simulink model "JSON_TEST_2022"  (R2022a)
settings: Solver=VariableStepAuto  StartTime=0.0  StopTime=10.0  RelTol=1e-3
libraries: dspnetwork x1, instrumentlib x1
settings Model: Creator=santh  LastModifiedBy=santh
settings ModelReferenceCC: EnableRefExpFcnMdlSchedulingChecks=off
settings RTWCC: Description=Generic Real-Time Target  GPUComputeCapability=5.0

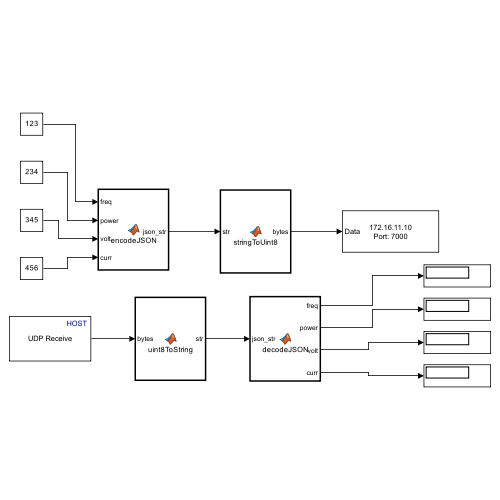
[thumbnail: Simulink's stored preview of the top-level diagram]
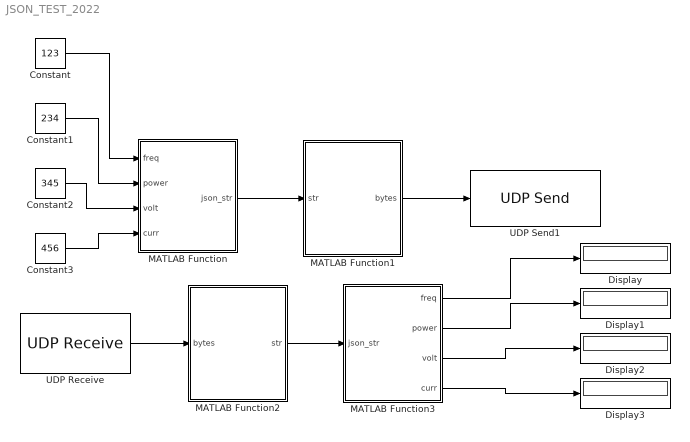
== system JSON_TEST_2022 ==
  Constant : Constant  Value=123
  Constant1 : Constant  Value=234
  Constant2 : Constant  Value=345
  Constant3 : Constant  Value=456
  Display{,1..3} (4 alike) : Display
  MATLAB Function : MATLAB Function  TreatAsAtomicUnit=on
  MATLAB Function1 : MATLAB Function  TreatAsAtomicUnit=on
  MATLAB Function2 : MATLAB Function  TreatAsAtomicUnit=on
  MATLAB Function3 : MATLAB Function  TreatAsAtomicUnit=on
  UDP Receive : dspnetwork/UDP Receive  localURL='0.0.0.0'  localPort=7000  remoteURL='172.16.11.10'  remotePort=-1  recvBufferSize=30  dims=64  signalDatatype=uint8  isComplex=off  isVarSize=on  showBlockingTime=on  blockingTime=0  sampletime=0.01  blockPlatform=HOST
  UDP Send1 : instrumentlib/UDP Send  Host=172.16.11.10  Port=7000  LocalAddress=176.16.11.69  LocalPort=7000  EnablePortSharing=off  OutputDatagramPacketSize=20  ByteOrder=BigEndian  EnableBlockingMode=on
  wires:
  Constant/1 -> MATLAB Function/1(freq)
  Constant1/1 -> MATLAB Function/2(power)
  Constant2/1 -> MATLAB Function/3(volt)
  Constant3/1 -> MATLAB Function/4(curr)
  MATLAB Function/1(json_str) -> MATLAB Function1/1(str)
  MATLAB Function1/1(bytes) -> UDP Send1/1
  UDP Receive/1 -> MATLAB Function2/1(bytes)
  MATLAB Function2/1(str) -> MATLAB Function3/1(json_str)
  MATLAB Function3/1(freq) -> Display/1
  MATLAB Function3/2(power) -> Display1/1
  MATLAB Function3/3(volt) -> Display2/1
  MATLAB Function3/4(curr) -> Display3/1

== matlab function JSON_TEST_2022/MATLAB Function1 ==
  data: str input; bytes output
function bytes = stringToUint8(str)
    bytes = uint8(char(str));
end

== matlab function JSON_TEST_2022/MATLAB Function ==
  data: freq input; json_str output; power input; volt input; curr input
function json_str = encodeJSON(freq, power, volt, curr)
    data = struct('frequency', freq, 'power', power, 'voltage', volt, 'current', curr);
    json_str = jsonencode(data);
end

== matlab function JSON_TEST_2022/MATLAB Function2 ==
  data: bytes input; str output
function str = uint8ToString(bytes)
    % Convert uint8 vector to string, removing trailing nulls
    str = char(bytes(bytes ~= 0));
end

== matlab function JSON_TEST_2022/MATLAB Function3 ==
  data: json_str input; freq output; power output; volt output; curr output
function [freq, power, volt, curr] = decodeJSON(json_str)
    % Decode JSON string and extract four parameters
    try
        data = jsondecode(json_str);
        freq = data.frequency;
        power = data.power;
        volt = data.voltage;
        curr = data.current;
    catch e
        % Handle JSON decoding errors
        disp(['JSON decode error: ', e.message]);
        freq = 0.0;
        power = 0.0;
        volt = 0.0;
        curr = 0.0;
    end
end
